simulink model "Aufgabe4_Bausteine"  (R2016a)
settings: Solver=ode45  StartTime=0.0  StopTime=10.0  RelTol=1e-3
undefined symbols (not defined in the file): magnitude, N, Tbit5_0
libraries: dspstat3 x2, commdigbbndam3 x1, simulink_extras x1, commsink2 x1, NoiseLib_2019 x1, Rectfilter_2012 x1
settings Model: Creator=Bornitz  LastModifiedBy=Bornitz
settings DataIOCC: LimitDataPoints=on  SaveFormat=Array  SignalLoggingSaveFormat=ModelDataLogs
settings OptimizationCC: ExpressionDepthLimit=2147483647
settings DebuggingCC: UnderspecifiedInitializationDetection=Classic  MergeDetectMultiDrivingBlocksExec=none  SolverPrmCheckMsg=warning  MultiTaskDSMMsg=warning  MultiTaskCondExecSysMsg=none  FcnCallInpInsideContextMsg=UseLocalSettings  StateNameClashWarn=warning  StrictBusMsg=None
settings HardwareCC: ProdBitPerPointer=32  ProdLargestAtomicFloat=None  ProdIntDivRoundTo=Undefined  ProdEndianess=Unspecified  ProdWordSize=32  ProdHWDeviceType=32-bit Generic
settings ModelReferenceCC: PropagateSignalLabelsOutOfModel=off
settings GRTTargetCC: CombineOutputUpdateFcns=off  GRTInterface=on
settings ConfigComp: CovModelRefEnable=Off

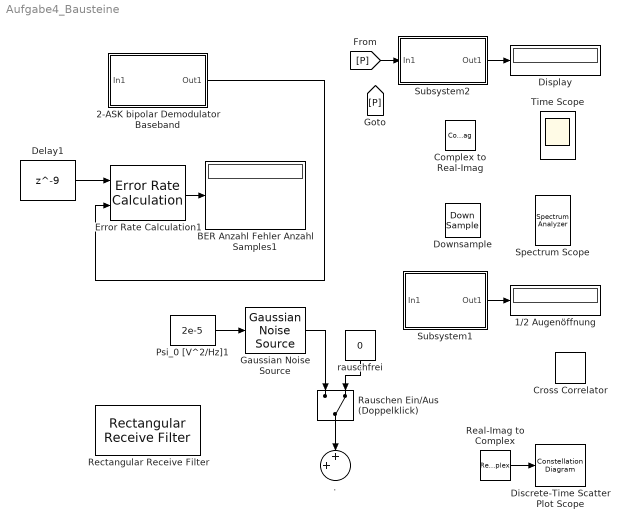
== system Aufgabe4_Bausteine ==
  . : Sum  Inputs=++|  SampleTime=Tbit5_0/16
  1/2 Augenöffnung : Display
  2-ASK bipolar Demodulator Baseband : Subsystem
      mask Display:
      | plot(0,0,100,100,[20+1.5*[[0:.8:10] [10:1.6:20] [20:.8:30]] 65 65 65 65+10*[0 1 1 2 2 3]],[85+10*[sin([0:.8:10]*pi*2/5) sin([10:1.6:20]*pi/5) sin([20:.8:30]*pi*2/5)] 85 99 75 85+8*[1 1 -1 -1 1 1]]);
      | disp('\nGeneral\nASK-Demodulator')
  BER Anzahl Fehler Anzahl Samples1 : Display
      settings: Format=short_e
  Complex to Real-Imag : ComplexToRealImag  Output=Real
  Cross Correlator : simulink_extras/Additional Sinks/Cross Correlator  npts=100  HowOften=50  sampleT=0.0002
  Delay1 : Delay  DelayLength=9  InitialCondition=0  InputProcessing=Columns as channels (frame based)
  Discrete-Time Scatter Plot Scope : ConstellationDiagram  Tag=ScatterPlot
  Display : Display
  Downsample : DownSample  N=N  RateOptions=Allow multirate processing
  Error Rate Calculation1 : commsink2/Error Rate Calculation  N=0  st_delay=800  cp_mode=Entire frame  subframe=1  PMode=Port  WsName=ErrorVec  RsMode2=off  stop=off  numErr=100  maxBits=1e6
  Gaussian Noise Source : NoiseLib_2019/Gaussian Noise Source  SystemSampleTime=-1
  Psi_0 [V^2/Hz]1 : Constant  Value=2e-5
  Rauschen Ein/Aus (Doppelklick) : ManualSwitch  CurrentSetting=0
  Real-Imag to Complex : RealImagToComplex  Input=Real
  Rectangular Receive Filter : Rectfilter_2012/Rectangular Receive Filter  N=N
  Spectrum Scope : SpectrumAnalyzer
  Subsystem1 : Subsystem
      mask Display:
      | image('openeye1.bmp',[0.1 0.3 0.8 0.57])
      | disp('\n\n\nAugenöffnung')
  Subsystem2 : Subsystem
      mask Display: disp('Leistungs-\n messung')
  Time Scope : Scope
  rauschfrei : Constant  Value=0
  wires:
  Real-Imag to Complex/1 -> Discrete-Time Scatter Plot Scope/1
  rauschfrei/1 -> Rauschen Ein/Aus (Doppelklick)/2
  Gaussian Noise Source/1 -> Rauschen Ein/Aus (Doppelklick)/1
  Rauschen Ein/Aus (Doppelklick)/1 -> ./1
  Psi_0 [V^2/Hz]1/1 -> Gaussian Noise Source/1
  Subsystem1/1(Out1) -> 1/2 Augenöffnung/1
  Error Rate Calculation1/1 -> BER Anzahl Fehler Anzahl Samples1/1
  Delay1/1 -> Error Rate Calculation1/1
  2-ASK bipolar Demodulator Baseband/1(Out1) -> Error Rate Calculation1/2
  [P] -> Subsystem2/1(In1)
  Subsystem2/1(Out1) -> Display/1

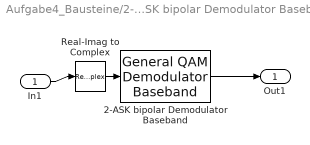
== system Aufgabe4_Bausteine/2-ASK bipolar Demodulator Baseband ==
  In1 : Inport
  2-ASK bipolar Demodulator Baseband : commdigbbndam3/General QAM Demodulator Baseband  SigCon=sigdem2  OutType=Bit  DecType=Hard decision  VarSource=Dialog  Variance=1  outDtypeBit=Inherit via internal rule  outDtype=Inherit via internal rule  roundingMode=Floor  overflowMode=Wrap  OvFlMode=off  OvFlModeLastStrValue=off  sigConstWordLen=16  sigConstDataTypeStr=Inherit: Same word length as input  sigConstLastDataTypeStr=Inherit: Same word length as input  accum1WordLen=32  accum1FracLen=30  prodInWordLen=32  prodInFracLen=30  prodInDataTypeStr=Inherit: Same as accumulator 1  prodInLastDataTypeStr=Inherit: Same as accumulator 1  prodOutWordLen=32  prodOutFracLen=30  accum2WordLen=32  accum2FracLen=30  accum3WordLen=32  accum3FracLen=30  nsiWordLen=32  nsiFracLen=30  nsiDataTypeStr=Inherit: Same as accumulator 3  nsiLastDataTypeStr=Inherit: Same as accumulator 3  invn0WordLen=16  invn0FracLen=8  invn0DataTypeStr=Inherit: Same word length as input  invn0LastDataTypeStr=Inherit: Same word length as input  outputWordLen=32  outputFracLen=30
  Real-Imag to Complex : RealImagToComplex  Input=Real
  Out1 : Outport
  wires:
  Real-Imag to Complex/1 -> 2-ASK bipolar Demodulator Baseband/1
  In1/1 -> Real-Imag to Complex/1
  2-ASK bipolar Demodulator Baseband/1 -> Out1/1

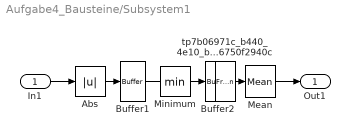
== system Aufgabe4_Bausteine/Subsystem1 ==
  In1 : Inport
  Abs : Abs
  Buffer1 : Buffer  N=20  V=4  TreatMby1Signals=One channel  OutputFrames=off
  Buffer2 : Buffer  N=20  V=4  TreatMby1Signals=One channel
  Mean : dspstat3/Mean  run=off  reset_popup=None  InputProcessing=Columns as channels (frame based)  directionMode=Each column  dimension=1  roiEnable=off  roiType=Rectangles  roiPortion=Entire ROI  roiOutput=Individual statistics for each ROI  roiFlag=off  outputDataTypeStr=Inherit: Same as accumulator  outputLastDataTypeStr=Inherit: Same as accumulator  outputMin=[]  outputMax=[]  roundingMode=Floor  overflowMode=off
  Minimum : MinMax
  tp7b06971c_b440_4e10_b14a_3b6750f2940c : FrameConversion  InheritSamplingMode=off
  Out1 : Outport
  wires:
  tp7b06971c_b440_4e10_b14a_3b6750f2940c/1 -> Minimum/1
  Buffer1/1 -> tp7b06971c_b440_4e10_b14a_3b6750f2940c/1
  Abs/1 -> Buffer1/1
  Minimum/1 -> Buffer2/1
  Buffer2/1 -> Mean/1
  In1/1 -> Abs/1
  Mean/1 -> Out1/1

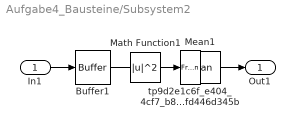
== system Aufgabe4_Bausteine/Subsystem2 ==
  In1 : Inport
  Buffer1 : Buffer  N=5000  TreatMby1Signals=One channel  OutputFrames=off
  Math Function1 : Math  Operator=magnitude^2  SaturateOnIntegerOverflow=on
  Mean1 : dspstat3/Mean  run=off  reset_popup=None  InputProcessing=Columns as channels (frame based)  directionMode=Each column  dimension=1  roiEnable=off  roiType=Rectangles  roiPortion=Entire ROI  roiOutput=Individual statistics for each ROI  roiFlag=off  outputDataTypeStr=Inherit: Same as accumulator  outputLastDataTypeStr=Inherit: Same as accumulator  outputMin=[]  outputMax=[]  roundingMode=Floor  overflowMode=off
  tp9d2e1c6f_e404_4cf7_b8ac_f8fd446d345b : FrameConversion  InheritSamplingMode=off
  Out1 : Outport
  wires:
  tp9d2e1c6f_e404_4cf7_b8ac_f8fd446d345b/1 -> Math Function1/1
  Buffer1/1 -> tp9d2e1c6f_e404_4cf7_b8ac_f8fd446d345b/1
  Mean1/1 -> Out1/1
  In1/1 -> Buffer1/1
  Math Function1/1 -> Mean1/1
